simulink model "taller5"  (R2025b)
settings: Solver=ode4  StartTime=0.0  StopTime=0.25  FixedStep=0.000001  RelTol=1e-3
values from neighbouring files (symbols this model uses):
  den = [1 2 3]    [taller2.m]    (also in taller5rlc.m = [1 R/L 1/(L*Cap)])
  K = 100    [taller5rlc.m]
  Kd = 0.10521281880029    (= 0.1052128188)    [taller5rlc.m]    (also in taller6.m; taller6e.m)
  Ki = 18678.6278431285    (= 18678.6278431)    [taller5rlc.m]    (also in taller6.m; taller6e.m)
  Kp = 89.0609480606665    (= 89.0609480607)    [taller5rlc.m]    (also in taller6.m; taller6e.m)
  num = 3    [taller2.m]    (also in taller5rlc.m = 45454.5454545)
libraries: slpidlib x1

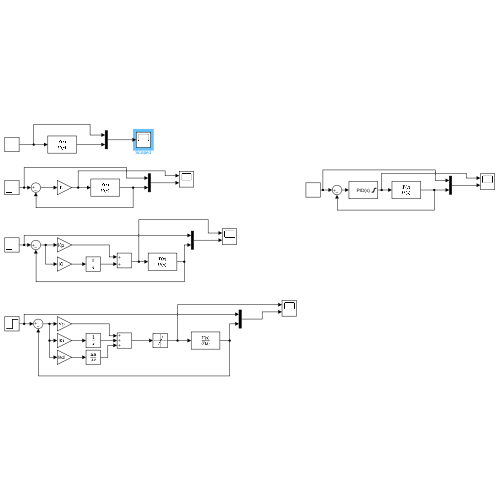
[thumbnail: Simulink's stored preview of the top-level diagram]
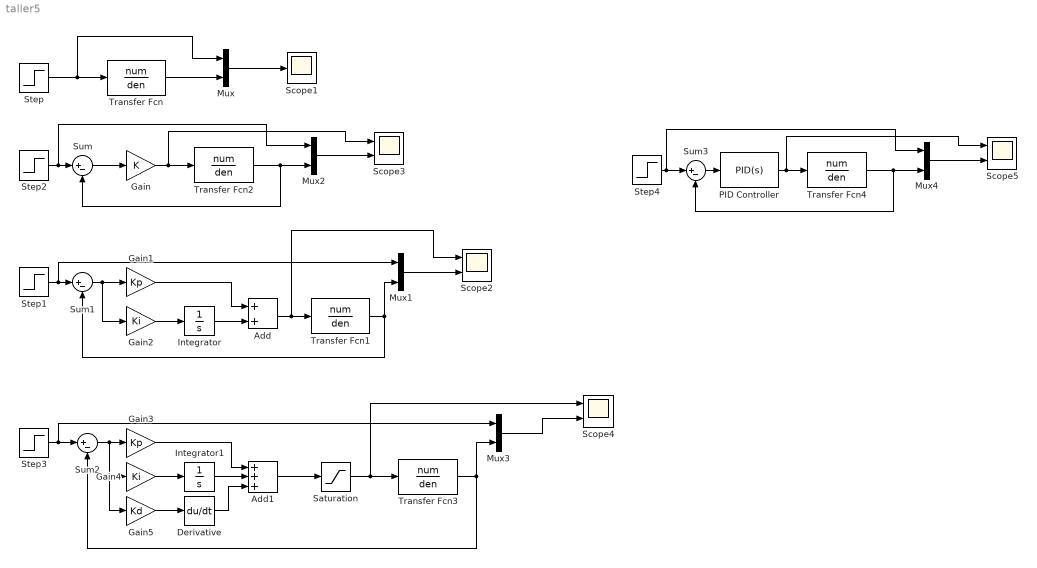
== system taller5 ==
  Add : Sum
  Add1 : Sum  Inputs=+++
  Derivative : Derivative
  Gain : Gain  Gain=K
  Gain1 : Gain  Gain=Kp
  Gain2 : Gain  Gain=Ki
  Gain3 : Gain  Gain=Kp
  Gain4 : Gain  Gain=Ki
  Gain5 : Gain  Gain=Kd
  Integrator : Integrator
  Integrator1 : Integrator
  Mux{,1..4} (5 alike) : Mux  Inputs=2
  PID Controller : slpidlib/PID Controller  Controller=PID  Form=Parallel  TimeDomain=Continuous-time  UseExternalTs=off  SampleTime=-1  IntegratorMethod=Forward Euler  FilterMethod=Forward Euler  ControllerParametersSource=internal  P=20  I=600  UseKiTs=off  D=0.03  UseExternalDerivativeSource=off  N=1000000  UseFilter=on  TunerSelectOption=Transfer Function Based (PID Tuner App)  InitialConditionSource=internal  InitialConditionForIntegrator=0  InitialConditionForFilter=0  DifferentiatorICPrevScaledInput=0  ExternalReset=none  TrackingMode=off  Kt=1  LimitOutput=on  SatLimitsSource=internal  UpperSaturationLimit=15  LowerSaturationLimit=-15  LinearizeAsGain=off  AntiWindupMode=none  Kb=1  LimitIntegrator=on  UpperIntegratorSaturationLimit=15  LowerIntegratorSaturationLimit=-15  POutMin=[]  POutMax=[]  IOutMin=[]  IOutMax=[]  DOutMin=[]  DOutMax=[]  NOutMin=[]  NOutMax=[]  SumOutMin=[]  SumOutMax=[]  SaturationOutMin=[]  SaturationOutMax=[]  PParamMin=[]  PParamMax=[]  IParamMin=[]  IParamMax=[]  DParamMin=[]  DParamMax=[]  NParamMin=[]  NParamMax=[]  KbParamMin=[]  KbParamMax=[]  KtParamMin=[]  KtParamMax=[]  KbOutMin=[]  KbOutMax=[]  KtOutMin=[]  KtOutMax=[]  IntegratorOutMin=[]  IntegratorOutMax=[]  FilterOutMin=[]  FilterOutMax=[]  SumI1OutMin=[]  SumI1OutMax=[]  SumI2OutMin=[]  SumI2OutMax=[]  SumI3OutMin=[]  SumI3OutMax=[]  SumI4OutMin=[]  SumI4OutMax=[]  SumDOutMin=[]  SumDOutMax=[]  DifferentiatorOutMin=[]  DifferentiatorOutMax=[]  FilterDiffOutCoefMin=[]  FilterDiffOutCoefMax=[]  ReciprocalOutMin=[]  ReciprocalOutMax=[]  SumDenOutMin=[]  SumDenOutMax=[]  SumNumOutMin=[]  SumNumOutMax=[]  DivideOutMin=[]  DivideOutMax=[]  UdiffTsProdOutMin=[]  UdiffTsProdOutMax=[]  NTsProdOutMin=[]  NTsProdOutMax=[]  UintegralTsProdOutMin=[]  UintegralTsProdOutMax=[]  UngainTsProdOutMin=[]  UngainTsProdOutMax=[]  ClampingZeroOutDataTypeStr=Inherit: Inherit via back propagation  ClampingZeroOutMin=[]  ClampingZeroOutMax=[]  FilterDenConstantOutDataTypeStr=Inherit: Inherit via back propagation  FilterDenConstantOutMin=[]  FilterDenConstantOutMax=[]  PCopyOutDataTypeStr=Inherit: Inherit via back propagation  PCopyOutMin=[]  PCopyOutMax=[]  NCopyOutDataTypeStr=Inherit: Inherit via back propagation  NCopyOutMin=[]  NCopyOutMax=[]  IntegratorContinuousStateAttributes=''  IntegratorStateMustResolveToSignalObject=off  IntegratorRTWStateStorageClass=Auto  FilterContinuousStateAttributes=''  FilterStateMustResolveToSignalObject=off  FilterRTWStateStorageClass=Auto  ParallelPVariant=InternalParameters  IdealPVariant=Disabled  IVariant=InternalParameters  DVariant=InternalParameters  IntegratorVariant=Continuous  SatVariant=Enabled  AWVariant=Passthrough  PCopyVariant=Disabled  TRVariant=Disabled  FdbkBlocksVariant=Forward  IdealPFdbkVariant=Disabled  SatFdbkVariant=Disabled  DerivativeFilterVariant=ContFilter  NVariant=InternalParameters  NCopyVariant=Disabled  FilterICVariant=InternalICsFilter  IntegratorICVariant=InternalICs  ExternalResetVariant=Disabled  TRSumVariant=Passthrough  SumFdbkVariant=Disabled  SumVariant=Sum_PID  TsampFilterVariant=InternalTs  TsampNgainVariant=Passthrough  TsampIntegralVariant=Disabled_SignalSpec  ExternalSaturationOutDataTypeStr=Inherit: Same as second input  DerivativeSourceVariant=ErrorSignal  PreIntVariant=InternalPreInt
  Saturation : Saturate  UpperLimit=15  LowerLimit=-15
  Scope1 : Scope
      settings: ActiveDisplayYMinimum=-1.0563018488665101  ActiveDisplayYMaximum=9.5067166397985936
  Scope{2..5} (4 alike) : Scope  NumInputPorts=2
      Scope2 settings: ActiveDisplayYMinimum=-46.886023861196747  ActiveDisplayYMaximum=60.857706354947787
      Scope3 settings: ActiveDisplayYMinimum=-0.62499999999999989  ActiveDisplayYMaximum=5.625  DataLoggingVariableName=ScopeData2
      Scope4 settings: ActiveDisplayYMinimum=-18.75  ActiveDisplayYMaximum=18.75  DataLoggingVariableName=ScopeData3
      Scope5 settings: ActiveDisplayYMinimum=-5.2082407847616192  ActiveDisplayYMaximum=17.245360087195735  DataLoggingVariableName=ScopeData4
  Step{,1..3} (4 alike) : Step  Time=0.01  After=5  SampleTime=0
  Step4 : Step  Time=0.01  SampleTime=0
  Sum{,1..3} (4 alike) : Sum  Inputs=|+-
  Transfer Fcn{,1..2,4} (4 alike) : TransferFcn  Numerator=num  Denominator=den
  Transfer Fcn3 : TransferFcn  Numerator=num  Denominator=den  AbsoluteTolerance=0.0001
  wires:
  Step/1 -> Mux/1, Transfer Fcn/1
  Transfer Fcn/1 -> Mux/2
  Mux/1 -> Scope1/1
  Transfer Fcn2/1 -> Sum/2, Mux2/2
  Mux2/1 -> Scope3/2
  Gain/1 -> Scope3/1, Transfer Fcn2/1
  Sum/1 -> Gain/1
  Step2/1 -> Mux2/1, Sum/1
  Transfer Fcn1/1 -> Mux1/2, Sum1/2
  Sum1/1 -> Gain2/1, Gain1/1
  Mux1/1 -> Scope2/2
  Gain1/1 -> Add/1
  Step1/1 -> Mux1/1, Sum1/1
  Gain2/1 -> Integrator/1
  Integrator/1 -> Add/2
  Add/1 -> Scope2/1, Transfer Fcn1/1
  Gain4/1 -> Integrator1/1
  Sum2/1 -> Gain3/1, Gain5/1, Gain4/1
  Transfer Fcn3/1 -> Mux3/2, Sum2/2
  Mux3/1 -> Scope4/2
  Gain3/1 -> Add1/1
  Integrator1/1 -> Add1/2
  Add1/1 -> Saturation/1
  Step3/1 -> Mux3/1, Sum2/1
  Gain5/1 -> Derivative/1
  Derivative/1 -> Add1/3
  Mux4/1 -> Scope5/2
  PID Controller/1 -> Scope5/1, Transfer Fcn4/1
  Transfer Fcn4/1 -> Sum3/2, Mux4/2
  Sum3/1 -> PID Controller/1
  Saturation/1 -> Scope4/1, Transfer Fcn3/1
  Step4/1 -> Mux4/1, Sum3/1
